simulink model "DcMotorControlSimscape"  (R2019b)
settings: Solver=VariableStepAuto  StartTime=0.0  StopTime=10.0  RelTol=1e-3  AbsTol=1e-3
libraries: fl_lib x15, nesl_utility x15, ee_lib x3
settings Model: Creator=fhasan1  LastModifiedBy=fhasan1
settings SolverCC: AutoScaleAbsTol=off
settings DebuggingCC: SymbolicDimsDataTypeCodeGenerationDiagnostic=none
settings SFSimCC: CustomCodeUndefinedFunction=UseInterfaceOnly
settings SimscapeCC: SimscapeLogType=all  SimscapeLogSimulationStatistics=on  SimscapeLogDataHistory=10000

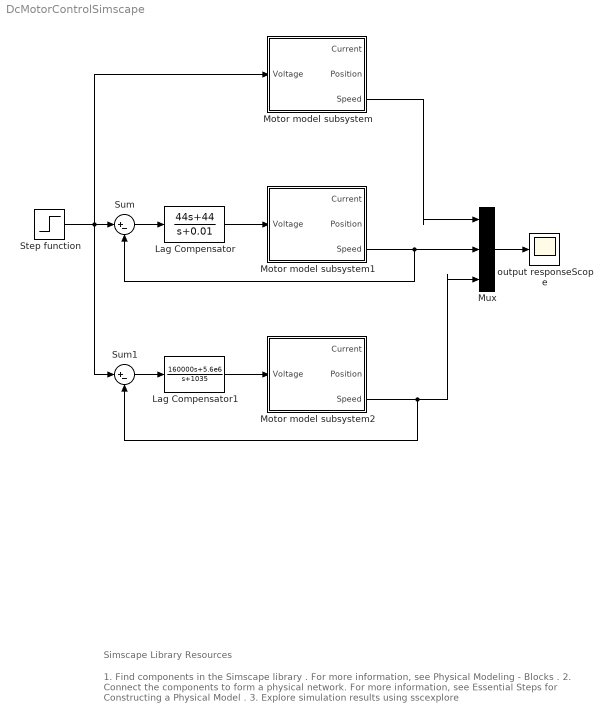
== system DcMotorControlSimscape ==
  note: 1. Find components in the Simscape library .
      | For more information, see Physical Modeling - Blocks .
      | 2. Connect the components to form a physical network.
      | For more information, see Essential Steps for Constructing a Physical Model .
      | 3. Explore simulation results using sscexplore
  note: Simscape Library Resources
  Lag Compensator : TransferFcn  Numerator=[44 44 ]  Denominator=[1 0.01 ]
  Lag Compensator1 : TransferFcn  Numerator=[160000 5.6e6 ]  Denominator=[1 1035 ]
  Motor model subsystem : Subsystem
  Motor model subsystem1 : Subsystem
  Motor model subsystem2 : Subsystem
  Mux : Mux  Inputs=3
  Step function : Step  Time=0  SampleTime=0
  Sum : Sum  Inputs=|+-
  Sum1 : Sum  Inputs=|+-
  "output responseScope " : Scope
  wires:
  Step function/1 -> Motor model subsystem/1(Voltage), Sum1/1, Sum/1
  Sum/1 -> Lag Compensator/1
  Sum1/1 -> Lag Compensator1/1
  Mux/1 -> "output responseScope "/1
  Lag Compensator1/1 -> Motor model subsystem2/1(Voltage)
  Motor model subsystem1/3(Speed) -> Sum/2, Mux/2
  Lag Compensator/1 -> Motor model subsystem1/1(Voltage)
  Motor model subsystem2/3(Speed) -> Mux/3, Sum1/2
  Motor model subsystem/3(Speed) -> Mux/1

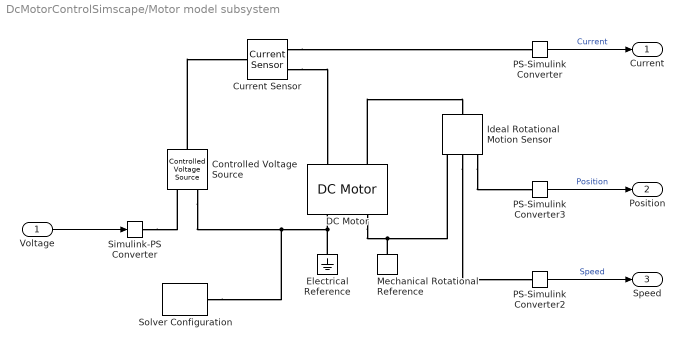
== system DcMotorControlSimscape/Motor model subsystem ==
  Voltage : Inport
  "Controlled Voltage Source " : fl_lib/Electrical/Electrical Sources/Controlled Voltage Source
  "Current Sensor " : fl_lib/Electrical/Electrical Sensors/Current Sensor
  "DC Motor " : ee_lib/Electromechanical/Brushed Motors/DC Motor  parameterization=1  Ra=1 Ohm  La=0.5 H  emf_or_torque=1  Kv=0.01 V/(rad/s)  Ki=6.876e-4 N*m/A  T_stall=0.24e-3 N*m  w_max=19100 rpm  w_rated=15000 rpm  P_rated=0.08 W  V_rated=1.5 V  J=0.01 kg*m^2  lam_param=1  lam=0.1 N*m/(rad/s)  i_noload=0 A  V_i_noload=1.5 V  speed0=0 rpm  alpha=3.93e-3 1/K  Tmeas=25 degC  thermal_mass=100 J/K  initial_temperature=25 degC
      settings: SourceProductName=Simscape Electrical
  Electrical Reference : fl_lib/Electrical/Electrical Elements/Electrical Reference
  "Ideal Rotational Motion Sensor " : fl_lib/Mechanical/Mechanical Sensors/Ideal Rotational Motion Sensor  offset=0 rad
  Mechanical Rotational Reference : fl_lib/Mechanical/Rotational Elements/Mechanical Rotational Reference
  "PS-Simulink Converter " : nesl_utility/PS-Simulink Converter  PhysicalDomain=network_engine_domain  SubClassName=ps_output  LeftPortType=input  RightPortType=output  PseudoPeriodic=off  Frequencies=[]  Unit=A  AffineConversion=off
  "PS-Simulink Converter2 " : nesl_utility/PS-Simulink Converter  PhysicalDomain=network_engine_domain  SubClassName=ps_output  LeftPortType=input  RightPortType=output  PseudoPeriodic=off  Frequencies=[]  Unit=rad/s  AffineConversion=off
  "PS-Simulink Converter3 " : nesl_utility/PS-Simulink Converter  PhysicalDomain=network_engine_domain  SubClassName=ps_output  LeftPortType=input  RightPortType=output  PseudoPeriodic=off  Frequencies=[]  Unit=rad  AffineConversion=off
  "Simulink-PS Converter " : nesl_utility/Simulink-PS Converter  PhysicalDomain=network_engine_domain  SubClassName=ps_input  LeftPortType=input  RightPortType=output  PseudoPeriodic=off  Frequencies=[]  NoiseDistribution=none  NoiseParameters=[]  Unit=V  AffineConversion=off  FilteringAndDerivatives=provide  SimscapeFilterOrder=1  InputFilterTimeConstant=0.001  UdotUserProvided=0
  "Solver Configuration " : nesl_utility/Solver Configuration  PhysicalDomain=network_engine_domain  SubClassName=solver  LeftPortType=input  RightPortType=generic  Tones=[]  Harmonics=[]  SimulateNoise=off  Profile=off  UseLocalSampling=off  EnableSwitchedLinearOptims=on  FrequencyDomain=off  UseCCode=off  RelTol=0.001  AbsTol=1e-06  MinStep=1e-09  ToWorkspace=off  RevertToSquareIcSolve=off  NumHomotopyIterations=100  PhasorMode=off  PhasorModeNumHarmonics=1  DoDC=off  ResidualTolerance=1e-09  UseLocalSolver=off  LocalSolverChoice=NE_BACKWARD_EULER_ADVANCER  LocalSolverSampleTime=0.001  DoFixedCost=off  MaxNonlinIter=3  MaxModeIter=2  LinearAlgebra=auto  EquationFormulation=NE_TIME_EF  DelaysMemoryBudget=1024  AutomaticFiltering=on  FilteringTimeConstant=0.001  PartitionStorageMethod=AS_NEEDED  PartitionMemoryBudget=1024  PartitionMethod=ROBUST
  Current : Outport
  Position : Outport  Port=2
  Speed : Outport  Port=3
  wires:
  "PS-Simulink Converter3 "/1 -> Position/1  "Position"
  "PS-Simulink Converter2 "/1 -> Speed/1  "Speed"
  Voltage/1 -> "Simulink-PS Converter "/1
  "PS-Simulink Converter "/1 -> Current/1  "Current"
  connections:
  "Controlled Voltage Source "/LConn1 -- "Current Sensor "/LConn1
  "Current Sensor "/RConn1 -- "PS-Simulink Converter "/LConn1
  "Simulink-PS Converter "/RConn1 -- "Controlled Voltage Source "/RConn1
  "Ideal Rotational Motion Sensor "/RConn2 -- "PS-Simulink Converter2 "/LConn1
  "Controlled Voltage Source "/RConn2 -- "Solver Configuration "/RConn1 -- Electrical Reference/LConn1 -- "DC Motor "/RConn1
  "Ideal Rotational Motion Sensor "/RConn3 -- "PS-Simulink Converter3 "/LConn1
  "DC Motor "/RConn2 -- Mechanical Rotational Reference/LConn1 -- "Ideal Rotational Motion Sensor "/RConn1
  "Current Sensor "/RConn2 -- "DC Motor "/LConn1
  "DC Motor "/LConn2 -- "Ideal Rotational Motion Sensor "/LConn1

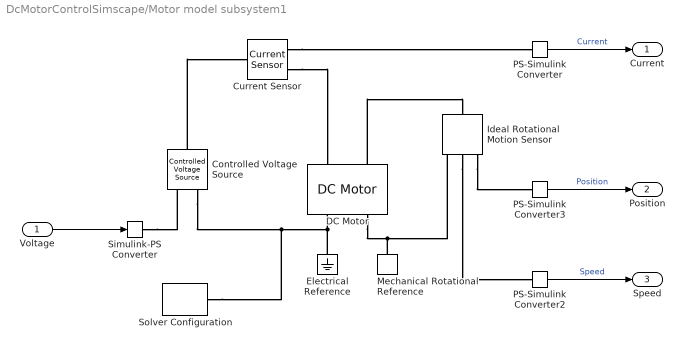
== system DcMotorControlSimscape/Motor model subsystem1 ==
  Voltage : Inport
  "Controlled Voltage Source " : fl_lib/Electrical/Electrical Sources/Controlled Voltage Source
  "Current Sensor " : fl_lib/Electrical/Electrical Sensors/Current Sensor
  "DC Motor " : ee_lib/Electromechanical/Brushed Motors/DC Motor  parameterization=1  Ra=1 Ohm  La=0.5 H  emf_or_torque=1  Kv=0.01 V/(rad/s)  Ki=6.876e-4 N*m/A  T_stall=0.24e-3 N*m  w_max=19100 rpm  w_rated=15000 rpm  P_rated=0.08 W  V_rated=1.5 V  J=0.01 kg*m^2  lam_param=1  lam=0.1 N*m/(rad/s)  i_noload=0 A  V_i_noload=1.5 V  speed0=0 rpm  alpha=3.93e-3 1/K  Tmeas=25 degC  thermal_mass=100 J/K  initial_temperature=25 degC
      settings: SourceProductName=Simscape Electrical
  Electrical Reference : fl_lib/Electrical/Electrical Elements/Electrical Reference
  "Ideal Rotational Motion Sensor " : fl_lib/Mechanical/Mechanical Sensors/Ideal Rotational Motion Sensor  offset=0 rad
  Mechanical Rotational Reference : fl_lib/Mechanical/Rotational Elements/Mechanical Rotational Reference
  "PS-Simulink Converter " : nesl_utility/PS-Simulink Converter  PhysicalDomain=network_engine_domain  SubClassName=ps_output  LeftPortType=input  RightPortType=output  PseudoPeriodic=off  Frequencies=[]  Unit=A  AffineConversion=off
  "PS-Simulink Converter2 " : nesl_utility/PS-Simulink Converter  PhysicalDomain=network_engine_domain  SubClassName=ps_output  LeftPortType=input  RightPortType=output  PseudoPeriodic=off  Frequencies=[]  Unit=rad/s  AffineConversion=off
  "PS-Simulink Converter3 " : nesl_utility/PS-Simulink Converter  PhysicalDomain=network_engine_domain  SubClassName=ps_output  LeftPortType=input  RightPortType=output  PseudoPeriodic=off  Frequencies=[]  Unit=rad  AffineConversion=off
  "Simulink-PS Converter " : nesl_utility/Simulink-PS Converter  PhysicalDomain=network_engine_domain  SubClassName=ps_input  LeftPortType=input  RightPortType=output  PseudoPeriodic=off  Frequencies=[]  NoiseDistribution=none  NoiseParameters=[]  Unit=V  AffineConversion=off  FilteringAndDerivatives=provide  SimscapeFilterOrder=1  InputFilterTimeConstant=0.001  UdotUserProvided=0
  "Solver Configuration " : nesl_utility/Solver Configuration  PhysicalDomain=network_engine_domain  SubClassName=solver  LeftPortType=input  RightPortType=generic  Tones=[]  Harmonics=[]  SimulateNoise=off  Profile=off  UseLocalSampling=off  EnableSwitchedLinearOptims=on  FrequencyDomain=off  UseCCode=off  RelTol=0.001  AbsTol=1e-06  MinStep=1e-09  ToWorkspace=off  RevertToSquareIcSolve=off  NumHomotopyIterations=100  PhasorMode=off  PhasorModeNumHarmonics=1  DoDC=off  ResidualTolerance=1e-09  UseLocalSolver=off  LocalSolverChoice=NE_BACKWARD_EULER_ADVANCER  LocalSolverSampleTime=0.001  DoFixedCost=off  MaxNonlinIter=3  MaxModeIter=2  LinearAlgebra=auto  EquationFormulation=NE_TIME_EF  DelaysMemoryBudget=1024  AutomaticFiltering=on  FilteringTimeConstant=0.001  PartitionStorageMethod=AS_NEEDED  PartitionMemoryBudget=1024  PartitionMethod=ROBUST
  Current : Outport
  Position : Outport  Port=2
  Speed : Outport  Port=3
  wires:
  "PS-Simulink Converter3 "/1 -> Position/1  "Position"
  "PS-Simulink Converter2 "/1 -> Speed/1  "Speed"
  Voltage/1 -> "Simulink-PS Converter "/1
  "PS-Simulink Converter "/1 -> Current/1  "Current"
  connections:
  "Controlled Voltage Source "/LConn1 -- "Current Sensor "/LConn1
  "Current Sensor "/RConn1 -- "PS-Simulink Converter "/LConn1
  "Simulink-PS Converter "/RConn1 -- "Controlled Voltage Source "/RConn1
  "Ideal Rotational Motion Sensor "/RConn2 -- "PS-Simulink Converter2 "/LConn1
  "Solver Configuration "/RConn1 -- "Controlled Voltage Source "/RConn2 -- "DC Motor "/RConn1 -- Electrical Reference/LConn1
  "Ideal Rotational Motion Sensor "/RConn3 -- "PS-Simulink Converter3 "/LConn1
  "Ideal Rotational Motion Sensor "/RConn1 -- "DC Motor "/RConn2 -- Mechanical Rotational Reference/LConn1
  "Current Sensor "/RConn2 -- "DC Motor "/LConn1
  "DC Motor "/LConn2 -- "Ideal Rotational Motion Sensor "/LConn1

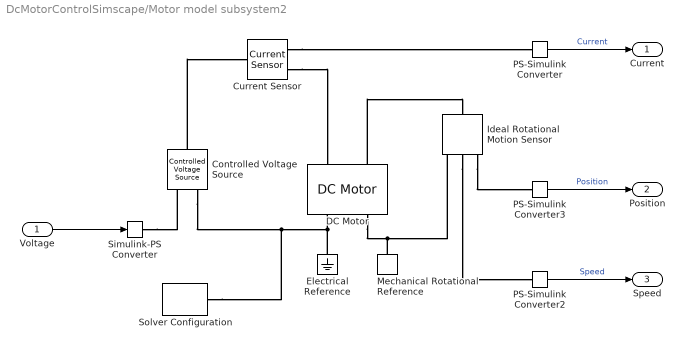
== system DcMotorControlSimscape/Motor model subsystem2 ==
  Voltage : Inport
  "Controlled Voltage Source " : fl_lib/Electrical/Electrical Sources/Controlled Voltage Source
  "Current Sensor " : fl_lib/Electrical/Electrical Sensors/Current Sensor
  "DC Motor " : ee_lib/Electromechanical/Brushed Motors/DC Motor  parameterization=1  Ra=1 Ohm  La=0.5 H  emf_or_torque=1  Kv=0.01 V/(rad/s)  Ki=6.876e-4 N*m/A  T_stall=0.24e-3 N*m  w_max=19100 rpm  w_rated=15000 rpm  P_rated=0.08 W  V_rated=1.5 V  J=0.01 kg*m^2  lam_param=1  lam=0.1 N*m/(rad/s)  i_noload=0 A  V_i_noload=1.5 V  speed0=0 rpm  alpha=3.93e-3 1/K  Tmeas=25 degC  thermal_mass=100 J/K  initial_temperature=25 degC
      settings: SourceProductName=Simscape Electrical
  Electrical Reference : fl_lib/Electrical/Electrical Elements/Electrical Reference
  "Ideal Rotational Motion Sensor " : fl_lib/Mechanical/Mechanical Sensors/Ideal Rotational Motion Sensor  offset=0 rad
  Mechanical Rotational Reference : fl_lib/Mechanical/Rotational Elements/Mechanical Rotational Reference
  "PS-Simulink Converter " : nesl_utility/PS-Simulink Converter  PhysicalDomain=network_engine_domain  SubClassName=ps_output  LeftPortType=input  RightPortType=output  PseudoPeriodic=off  Frequencies=[]  Unit=A  AffineConversion=off
  "PS-Simulink Converter2 " : nesl_utility/PS-Simulink Converter  PhysicalDomain=network_engine_domain  SubClassName=ps_output  LeftPortType=input  RightPortType=output  PseudoPeriodic=off  Frequencies=[]  Unit=rad/s  AffineConversion=off
  "PS-Simulink Converter3 " : nesl_utility/PS-Simulink Converter  PhysicalDomain=network_engine_domain  SubClassName=ps_output  LeftPortType=input  RightPortType=output  PseudoPeriodic=off  Frequencies=[]  Unit=rad  AffineConversion=off
  "Simulink-PS Converter " : nesl_utility/Simulink-PS Converter  PhysicalDomain=network_engine_domain  SubClassName=ps_input  LeftPortType=input  RightPortType=output  PseudoPeriodic=off  Frequencies=[]  NoiseDistribution=none  NoiseParameters=[]  Unit=V  AffineConversion=off  FilteringAndDerivatives=provide  SimscapeFilterOrder=1  InputFilterTimeConstant=0.001  UdotUserProvided=0
  "Solver Configuration " : nesl_utility/Solver Configuration  PhysicalDomain=network_engine_domain  SubClassName=solver  LeftPortType=input  RightPortType=generic  Tones=[]  Harmonics=[]  SimulateNoise=off  Profile=off  UseLocalSampling=off  EnableSwitchedLinearOptims=on  FrequencyDomain=off  UseCCode=off  RelTol=0.001  AbsTol=1e-06  MinStep=1e-09  ToWorkspace=off  RevertToSquareIcSolve=off  NumHomotopyIterations=100  PhasorMode=off  PhasorModeNumHarmonics=1  DoDC=off  ResidualTolerance=1e-09  UseLocalSolver=off  LocalSolverChoice=NE_BACKWARD_EULER_ADVANCER  LocalSolverSampleTime=0.001  DoFixedCost=off  MaxNonlinIter=3  MaxModeIter=2  LinearAlgebra=auto  EquationFormulation=NE_TIME_EF  DelaysMemoryBudget=1024  AutomaticFiltering=on  FilteringTimeConstant=0.001  PartitionStorageMethod=AS_NEEDED  PartitionMemoryBudget=1024  PartitionMethod=ROBUST
  Current : Outport
  Position : Outport  Port=2
  Speed : Outport  Port=3
  wires:
  "PS-Simulink Converter3 "/1 -> Position/1  "Position"
  "PS-Simulink Converter2 "/1 -> Speed/1  "Speed"
  Voltage/1 -> "Simulink-PS Converter "/1
  "PS-Simulink Converter "/1 -> Current/1  "Current"
  connections:
  "Controlled Voltage Source "/LConn1 -- "Current Sensor "/LConn1
  "Current Sensor "/RConn1 -- "PS-Simulink Converter "/LConn1
  "Simulink-PS Converter "/RConn1 -- "Controlled Voltage Source "/RConn1
  "Ideal Rotational Motion Sensor "/RConn2 -- "PS-Simulink Converter2 "/LConn1
  "Solver Configuration "/RConn1 -- "Controlled Voltage Source "/RConn2 -- "DC Motor "/RConn1 -- Electrical Reference/LConn1
  "Ideal Rotational Motion Sensor "/RConn3 -- "PS-Simulink Converter3 "/LConn1
  "Ideal Rotational Motion Sensor "/RConn1 -- "DC Motor "/RConn2 -- Mechanical Rotational Reference/LConn1
  "Current Sensor "/RConn2 -- "DC Motor "/LConn1
  "DC Motor "/LConn2 -- "Ideal Rotational Motion Sensor "/LConn1
